simulink model "model"  (R2016b)
settings: Solver=VariableStepAuto  StartTime=0.0  StopTime=12100  RelTol=1e-3
undefined symbols (not defined in the file): C1, C2, C3, DOD, DOD1, OCV, R0, R1, R2, R3, sigbuilder_block
settings Model: Creator=Karel Van Peteghem  LastModifiedBy=Karel Van Peteghem

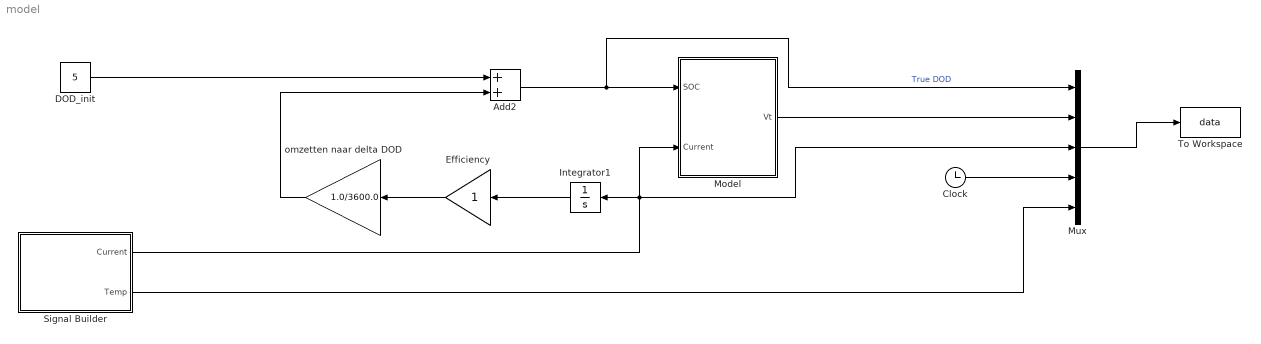
== system model ==
  Add2 : Sum
  Clock : Clock
  "DOD_init " : Constant  Value=5
  Efficiency : Gain
  Integrator1 : Integrator
  Model : Subsystem
  Mux : Mux  Inputs=5
  Signal Builder : Subsystem  Tag=STV Subsys  LoadFcn=sigbuilder_block('load');  StartFcn=sigbuilder_block('start');  StopFcn=sigbuilder_block('stop');  ClipboardFcn=sigbuilder_block('clipboard');  mask(Sigbuilder block){tuvar=[0:10]}
      mask help: Simulink:masks:SigbuilderBlock_MD
      mask init:
      | if ~strcmp(get_param(bdroot(gcbh),'SimulationStatus'),'stopped') tuvar = sigbuilder_block('maskInit'); end
      settings: CopyFcn=sigbuilder_block('copy');  DeleteFcn=sigbuilder_block('delete');  ModelCloseFcn=sigbuilder_block('modelClose');  PreSaveFcn=sigbuilder_block('preSave');  PauseFcn=sigbuilder_block('pause');  ContinueFcn=sigbuilder_block('continue');  NameChangeFcn=sigbuilder_block('namechange');  OpenFcn=sigbuilder_block('open',[228 111.75 550.5 359.25 ]);  CloseFcn=sigbuilder_block('close');
      mask Display: plot(0, 0, 100, 100,[2, 2, 32, 32, 2], [68, 8, 8, 68, 68],[32, 2], [38, 38], [32, 19, 2],[53, 60, 44], [32, 17, 17, 2],[16, 16, 31, 31]);txt = getActiveGroup(gcbh);text(2, 100, txt,'verticalAlignment', 'top');
  To Workspace : ToWorkspace  VariableName=data  SampleTime=1
  omzetten naar delta DOD : Gain  Gain=1.0/3600.0
  wires:
  Mux/1 -> To Workspace/1
  "DOD_init "/1 -> Add2/1
  Add2/1 -> Mux/1, Model/1(SOC)  "True DOD"
  Efficiency/1 -> omzetten naar delta DOD/1
  omzetten naar delta DOD/1 -> Add2/2
  Signal Builder/1(Current) -> Model/2(Current), Mux/3, Integrator1/1
  Integrator1/1 -> Efficiency/1
  Model/1(Vt) -> Mux/2
  Clock/1 -> Mux/4
  Signal Builder/2(Temp) -> Mux/5

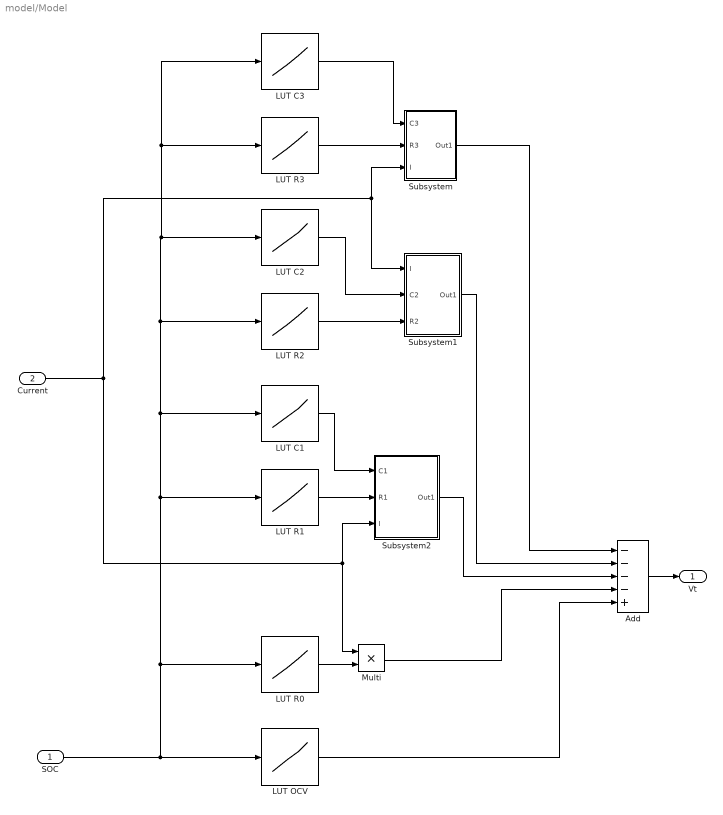
== system model/Model ==
  SOC : Inport
  Current : Inport  Port=2
  Add : Sum  Inputs=----+
  LUT C1 : Lookup_n-D  NumberOfTableDimensions=1  LookupTableObject=OCVaangepast  BreakpointsForDimension1=DOD1  Table=C1  InternalRulePriority=Speed  RndMeth=Simplest  InputSameDT=on
  "LUT C2 " : Lookup_n-D  NumberOfTableDimensions=1  LookupTableObject=OCVaangepast  BreakpointsForDimension1=DOD1  Table=C2  InternalRulePriority=Speed  RndMeth=Simplest  InputSameDT=on
  LUT C3 : Lookup_n-D  NumberOfTableDimensions=1  LookupTableObject=OCVaangepast  BreakpointsForDimension1=DOD1  Table=C3  InternalRulePriority=Speed  RndMeth=Simplest  InputSameDT=on
  LUT OCV : Lookup_n-D  NumberOfTableDimensions=1  LookupTableObject=OCVaangepast  BreakpointsForDimension1=DOD  Table=OCV  InternalRulePriority=Speed  RndMeth=Simplest  InputSameDT=on
  LUT R0 : Lookup_n-D  NumberOfTableDimensions=1  LookupTableObject=OCVaangepast  BreakpointsForDimension1=DOD1  Table=R0  InternalRulePriority=Speed  RndMeth=Simplest  InputSameDT=on
  LUT R1 : Lookup_n-D  NumberOfTableDimensions=1  LookupTableObject=OCVaangepast  BreakpointsForDimension1=DOD1  Table=R1  InternalRulePriority=Speed  RndMeth=Simplest  InputSameDT=on
  LUT R2 : Lookup_n-D  NumberOfTableDimensions=1  LookupTableObject=OCVaangepast  BreakpointsForDimension1=DOD1  Table=R2  InternalRulePriority=Speed  RndMeth=Simplest  InputSameDT=on
  LUT R3 : Lookup_n-D  NumberOfTableDimensions=1  LookupTableObject=OCVaangepast  BreakpointsForDimension1=DOD1  Table=R3  InternalRulePriority=Speed  RndMeth=Simplest  InputSameDT=on
  "Multi " : Product  Inputs=**
  Subsystem : Subsystem
  Subsystem1 : Subsystem
  Subsystem2 : Subsystem
  Vt : Outport
  wires:
  LUT C3/1 -> Subsystem/1("C3 ")
  LUT R3/1 -> Subsystem/2(R3)
  Add/1 -> Vt/1
  LUT OCV/1 -> Add/5
  LUT R1/1 -> Subsystem2/2(R1)
  LUT C1/1 -> Subsystem2/1(C1)
  Current/1 -> Subsystem2/3(I), "Multi "/1, Subsystem1/1(I), Subsystem/3(I)
  Subsystem2/1(Out1) -> Add/3
  Subsystem/1(Out1) -> Add/1
  Subsystem1/1(Out1) -> Add/2
  "Multi "/1 -> Add/4
  LUT R0/1 -> "Multi "/2
  LUT R2/1 -> Subsystem1/3(R2)
  SOC/1 -> LUT OCV/1, "LUT C2 "/1, LUT C3/1, LUT R3/1, LUT R2/1, LUT C1/1, LUT R1/1, LUT R0/1
  "LUT C2 "/1 -> Subsystem1/2("C2 ")

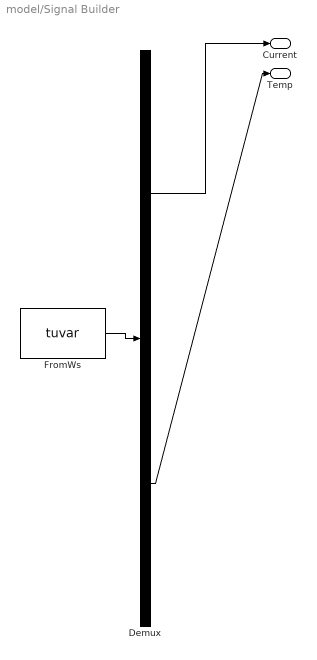
== system model/Signal Builder ==
  Demux : Demux  Tag=STV Demux  Outputs=2
  FromWs : FromWorkspace  Tag=STV FromWs  VariableName=tuvar  SampleTime=0
      SigBuilderData=|
      | common.afterFinalStr = 'Extrapolate'
      | common.sampleTime = 0
      | dataSet.timeRange = [0 12000]
      | dataSet.name = 'Blad1'
      | sbobj.Name = 'Signal Builder'
      | sbobj.Groups.Name = 'Blad1'
      | sbobj.Groups.Signals(1).Name = 'Current'
      | sbobj.Groups.Signals(1).XData = [0 100 100 1276 1276 12000]
      | sbobj.Groups.Signals(1).YData = [0 0 15 15 0 0]
      | sbobj.Groups.Signals(2).Name = 'Temp'
      | sbobj.Groups.Signals(2).XData = [0 100 1276 12000]
      | sbobj.Groups.Signals(2).YData = [25 25 25 25]
      | sbobj.Groups.TimeRange = [0 12000]
  Current : Outport  Tag=STV Outport
  Temp : Outport  Tag=STV Outport  Port=2
  wires:
  Demux/1 -> Current/1
  FromWs/1 -> Demux/1
  Demux/2 -> Temp/1

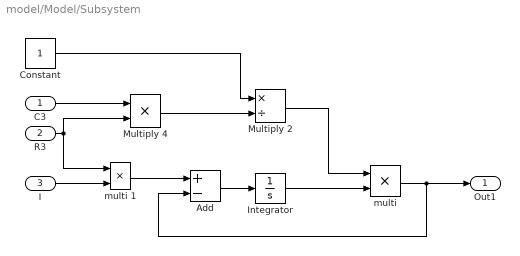
== system model/Model/Subsystem ==
  "C3 " : Inport
  R3 : Inport  Port=2
  I : Inport  Port=3
  Add : Sum  Inputs=+-
  Constant : Constant
  Integrator : Integrator
  Multiply 2 : Product  Inputs=*/
  Multiply 4 : Product  Inputs=**
  multi : Product  Inputs=**
  multi 1 : Product  Inputs=**
  Out1 : Outport
  wires:
  multi/1 -> Add/2, Out1/1
  Integrator/1 -> multi/2
  Constant/1 -> Multiply 2/1
  Multiply 2/1 -> multi/1
  Add/1 -> Integrator/1
  I/1 -> multi 1/2
  R3/1 -> Multiply 4/2, multi 1/1
  multi 1/1 -> Add/1
  "C3 "/1 -> Multiply 4/1
  Multiply 4/1 -> Multiply 2/2

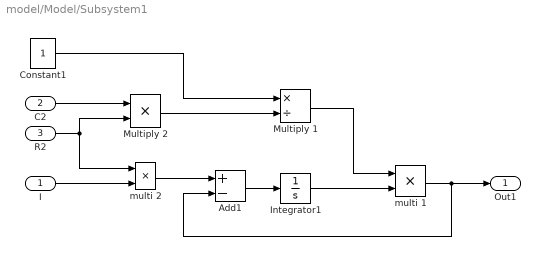
== system model/Model/Subsystem1 ==
  I : Inport
  "C2 " : Inport  Port=2
  R2 : Inport  Port=3
  Add1 : Sum  Inputs=+-
  Constant1 : Constant
  Integrator1 : Integrator
  Multiply 1 : Product  Inputs=*/
  Multiply 2 : Product  Inputs=**
  multi 1 : Product  Inputs=**
  multi 2 : Product  Inputs=**
  Out1 : Outport
  wires:
  multi 1/1 -> Out1/1, Add1/2
  Integrator1/1 -> multi 1/2
  Constant1/1 -> Multiply 1/1
  Multiply 1/1 -> multi 1/1
  Add1/1 -> Integrator1/1
  R2/1 -> Multiply 2/2, multi 2/1
  multi 2/1 -> Add1/1
  Multiply 2/1 -> Multiply 1/2
  I/1 -> multi 2/2
  "C2 "/1 -> Multiply 2/1

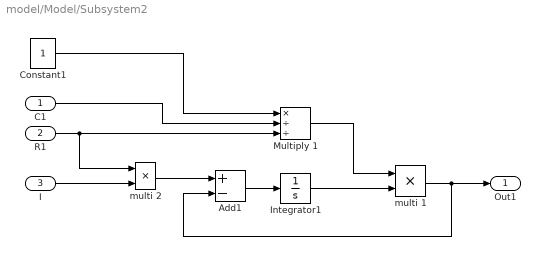
== system model/Model/Subsystem2 ==
  C1 : Inport
  R1 : Inport  Port=2
  I : Inport  Port=3
  Add1 : Sum  Inputs=+-
  Constant1 : Constant
  Integrator1 : Integrator
  Multiply 1 : Product  Inputs=*//
  multi 1 : Product  Inputs=**
  multi 2 : Product  Inputs=**
  Out1 : Outport
  wires:
  multi 1/1 -> Out1/1, Add1/2
  C1/1 -> Multiply 1/2
  Integrator1/1 -> multi 1/2
  Constant1/1 -> Multiply 1/1
  Multiply 1/1 -> multi 1/1
  Add1/1 -> Integrator1/1
  I/1 -> multi 2/2
  R1/1 -> multi 2/1, Multiply 1/3
  multi 2/1 -> Add1/1
